simulink model "TestFlightSim1D_g_m"  (R2020b)
settings: Solver=VariableStepAuto  StartTime=0.0  StopTime=85  RelTol=1e-10
settings Model: Creator=jonathan  LastModifiedBy=jonathan

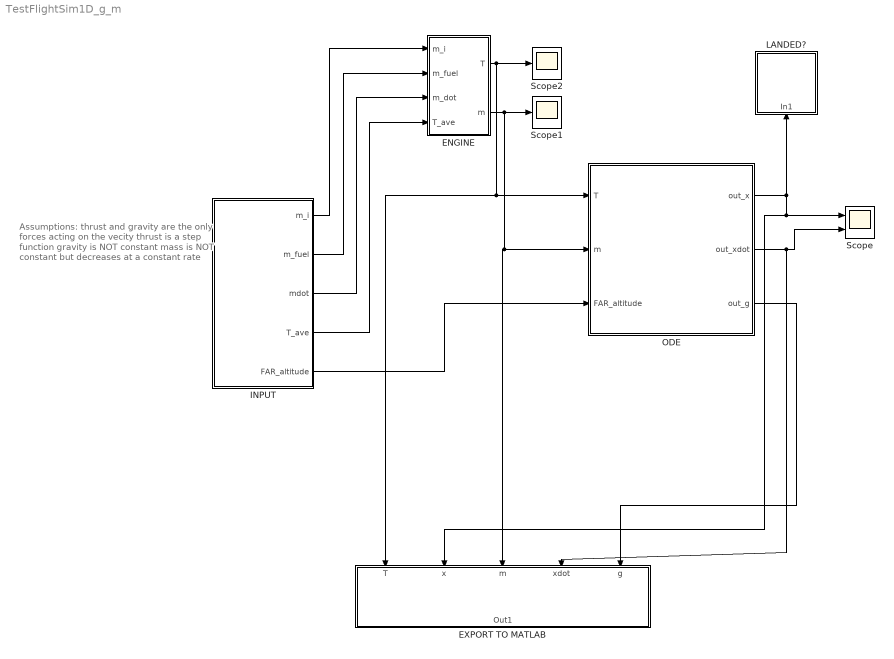
== system TestFlightSim1D_g_m ==
  note: Assumptions:
      | thrust and gravity are the only forces acting on the vecity
      | thrust is a step function
      | gravity is NOT constant
      | mass is NOT constant but decreases at a constant rate
  ENGINE : Subsystem
  EXPORT TO MATLAB : Subsystem
  INPUT : MATLAB Function  TreatAsAtomicUnit=on
  LANDED? : Subsystem
  ODE : Subsystem
  Scope : Scope  NumInputPorts=2
  Scope1 : Scope
  Scope2 : Scope
  wires:
  ODE/2(out_xdot) -> Scope/2, EXPORT TO MATLAB/4(xdot)
  ODE/1(out_x) -> Scope/1, EXPORT TO MATLAB/2(x), LANDED?/1(In1)
  INPUT/5(FAR_altitude) -> ODE/3(FAR_altitude)
  INPUT/4(T_ave) -> ENGINE/4(T_ave)
  INPUT/1(m_i) -> ENGINE/1(m_i)
  INPUT/2(m_fuel) -> ENGINE/2(m_fuel)
  INPUT/3(mdot) -> ENGINE/3(m_dot)
  ENGINE/1(T) -> ODE/1(T), EXPORT TO MATLAB/1(T), Scope2/1
  ENGINE/2(m) -> ODE/2(m), EXPORT TO MATLAB/3(m), Scope1/1
  ODE/3(out_g) -> EXPORT TO MATLAB/5(g)

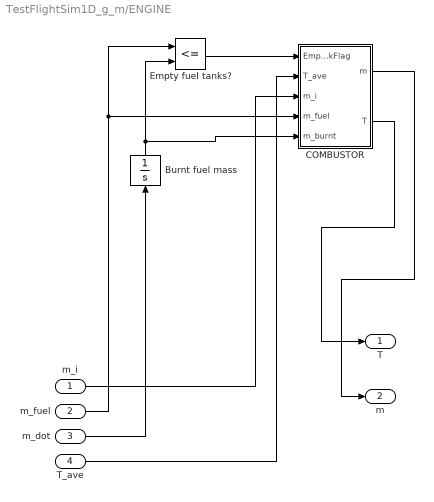
== system TestFlightSim1D_g_m/ENGINE ==
  m_i : Inport
  m_fuel : Inport  Port=2
  m_dot : Inport  Port=3
  T_ave : Inport  Port=4
  Burnt fuel mass : Integrator
  COMBUSTOR : MATLAB Function  TreatAsAtomicUnit=on
  Empty fuel tanks? : RelationalOperator  Operator=<=  OutDataTypeStr=boolean  RndMeth=Simplest
  T : Outport
  m : Outport  Port=2
  wires:
  COMBUSTOR/1(m) -> m/1
  T_ave/1 -> COMBUSTOR/2(T_ave)
  COMBUSTOR/2(T) -> T/1
  m_fuel/1 -> COMBUSTOR/4(m_fuel), Empty fuel tanks?/1
  m_dot/1 -> Burnt fuel mass/1
  Burnt fuel mass/1 -> Empty fuel tanks?/2, COMBUSTOR/5(m_burnt)
  m_i/1 -> COMBUSTOR/3(m_i)
  Empty fuel tanks?/1 -> COMBUSTOR/1(EmptyTankFlag)

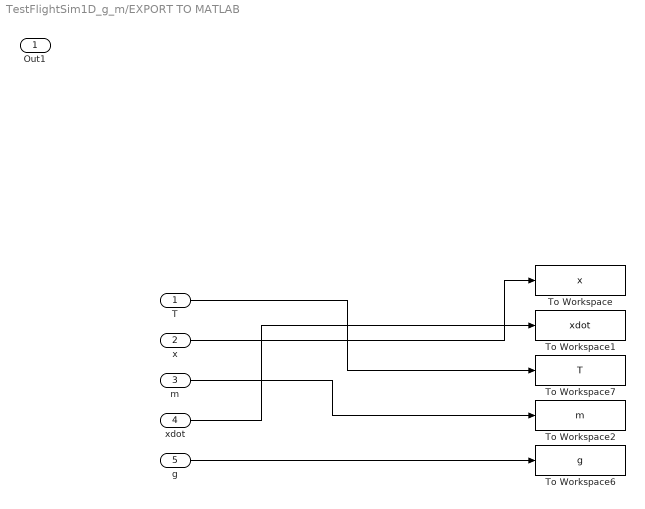
== system TestFlightSim1D_g_m/EXPORT TO MATLAB ==
  T : Inport
  x : Inport  Port=2
  m : Inport  Port=3
  xdot : Inport  Port=4
  g : Inport  Port=5
  To Workspace : ToWorkspace  VariableName=x  SaveFormat=Timeseries  SampleTime=-1
  To Workspace1 : ToWorkspace  VariableName=xdot  SaveFormat=Timeseries  SampleTime=-1
  To Workspace2 : ToWorkspace  VariableName=m  SaveFormat=Timeseries  SampleTime=-1
  To Workspace6 : ToWorkspace  VariableName=g  SaveFormat=Timeseries  SampleTime=-1
  To Workspace7 : ToWorkspace  VariableName=T  SaveFormat=Timeseries  SampleTime=-1
  Out1 : Outport
  wires:
  xdot/1 -> To Workspace1/1
  T/1 -> To Workspace7/1
  x/1 -> To Workspace/1
  m/1 -> To Workspace2/1
  g/1 -> To Workspace6/1

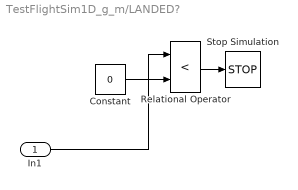
== system TestFlightSim1D_g_m/LANDED? ==
  In1 : Inport
  Constant : Constant  Value=0
  Relational Operator : RelationalOperator  Operator=<  OutDataTypeStr=boolean  RndMeth=Simplest
  Stop Simulation : Stop
  wires:
  In1/1 -> Relational Operator/1
  Constant/1 -> Relational Operator/2
  Relational Operator/1 -> Stop Simulation/1

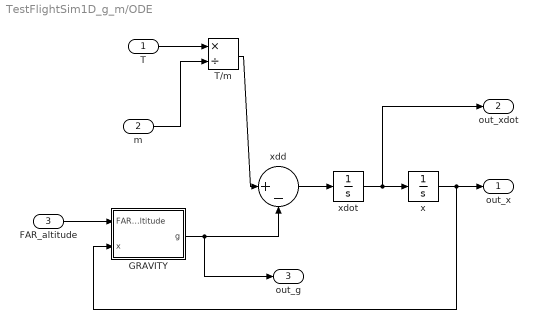
== system TestFlightSim1D_g_m/ODE ==
  T : Inport
  m : Inport  Port=2
  FAR_altitude : Inport  Port=3
  GRAVITY : MATLAB Function  TreatAsAtomicUnit=on
  T/m : Product  Inputs=*/
  x : Integrator
  xdd : Sum  Inputs=|+-
  xdot : Integrator
  out_x : Outport
  out_xdot : Outport  Port=2
  out_g : Outport  Port=3
  wires:
  m/1 -> T/m/2
  T/1 -> T/m/1
  x/1 -> GRAVITY/2(x), out_x/1
  xdot/1 -> out_xdot/1, x/1
  T/m/1 -> xdd/1
  xdd/1 -> xdot/1
  FAR_altitude/1 -> GRAVITY/1(FAR_altitude)
  GRAVITY/1(g) -> out_g/1, xdd/2

== matlab function TestFlightSim1D_g_m/ENGINE/COMBUSTOR ==
  data: m output; EmptyTankFlag input; T output; T_ave input; m_i input; m_fuel input; m_burnt input
function [m,T] = fcn(EmptyTankFlag, T_ave, m_i, m_fuel, m_burnt)
if EmptyTankFlag == 0
    T = T_ave;
    m = m_i - m_burnt;
else
    T = 0;
    m = m_i - m_fuel;
end

end

== matlab function TestFlightSim1D_g_m/INPUT ==
  data: m_i output; m_fuel output; mdot output; T_ave output; FAR_altitude output
function [m_i,m_fuel,mdot,T_ave,FAR_altitude] = fcn
% m_i - initial vehicle mass (assumed constant)
% m_fuel - fuel mass
% T_ave - average thrust
% ISP - specific impulse of engine
% FAR_altitude - altitude at FAR

m_i = 200*0.453592; % [kg]
m_fuel = 34*0.453592; % [kg]
T_ave = 880*4.45; % [N]
ISP = 230; % [kg]
FAR_altitude = 1068.0192; % [m] altitude of Ransburg, CA

% calculate mass flow rate
mdot = T_ave / (ISP * 9.8); % [kg/s]

end

== matlab function TestFlightSim1D_g_m/ODE/GRAVITY ==
  data: FAR_altitude input; g output; x input
function g = fcn(FAR_altitude,x)

RE = 6378e3; % [m] earth sea level radius
Mu_E = 3.986e14; % [m3/s2] gravitational parameter of earth

r = RE + FAR_altitude + x;

g = Mu_E*r^(-2);

end
